simulink model "p3"  (R2020b)
settings: Solver=VariableStepAuto  StartTime=0.0  StopTime=5  RelTol=1e-3
undefined symbols (not defined in the file): A, A1, B, B1, C, C1, K, K1, KDelay
libraries: simulink x2
settings Model: Creator=Julian  LastModifiedBy=Julian

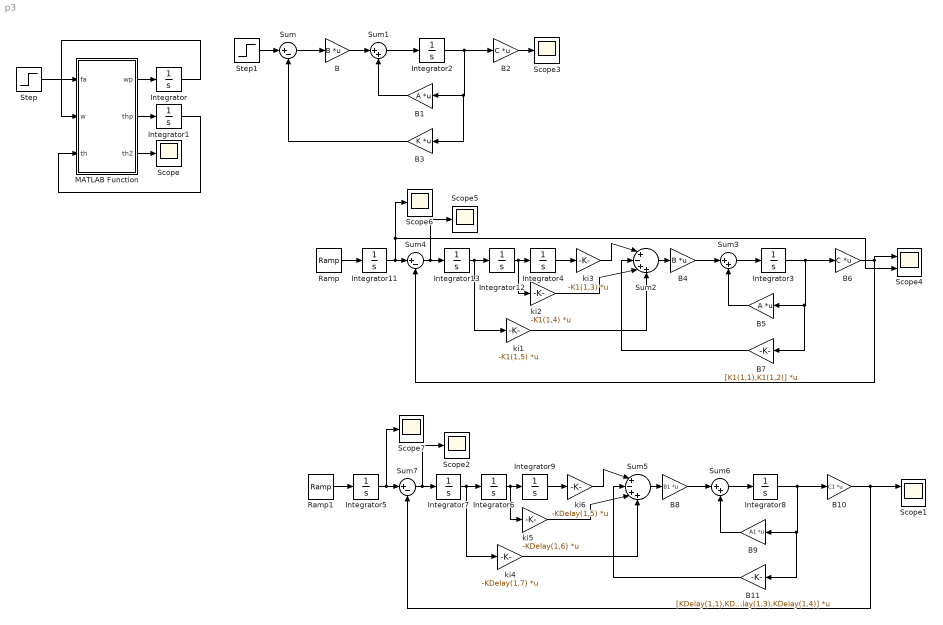
== system p3 ==
  B : Gain  Gain=B  Multiplication=Matrix(K*u)
  B1 : Gain  Gain=A  Multiplication=Matrix(K*u)
  B10 : Gain  Gain=C1  Multiplication=Matrix(K*u)
  B11 : Gain  Gain=[KDelay(1,1),KDelay(1,2),KDelay(1,3),KDelay(1,4)]  Multiplication=Matrix(K*u)
  B2 : Gain  Gain=C  Multiplication=Matrix(K*u)
  B3 : Gain  Gain=K  Multiplication=Matrix(K*u)
  B4 : Gain  Gain=B  Multiplication=Matrix(K*u)
  B5 : Gain  Gain=A  Multiplication=Matrix(K*u)
  B6 : Gain  Gain=C  Multiplication=Matrix(K*u)
  B7 : Gain  Gain=[K1(1,1),K1(1,2)]  Multiplication=Matrix(K*u)
  B8 : Gain  Gain=B1  Multiplication=Matrix(K*u)
  B9 : Gain  Gain=A1  Multiplication=Matrix(K*u)
  Integrator{,1..9,11..13} (13 alike) : Integrator
  MATLAB Function : MATLAB Function  TreatAsAtomicUnit=on
  Ramp : simulink/Sources/Ramp  slope=0.5  start=0  InitialOutput=0
  Ramp1 : simulink/Sources/Ramp  slope=0.5  start=0.5  InitialOutput=0
  Scope{,2..3,5..7} (6 alike) : Scope
  Scope1 : Scope  NumInputPorts=2
  Scope4 : Scope  NumInputPorts=2
  Step : Step  Time=0  SampleTime=0
  Step1 : Step  Time=0  SampleTime=0
  Sum : Sum  Inputs=|+-
  Sum1 : Sum  Inputs=|++
  Sum2 : Sum  Inputs=|+-++
  Sum3 : Sum  Inputs=|++
  Sum4 : Sum  Inputs=|+-
  Sum5 : Sum  Inputs=|+-++
  Sum6 : Sum  Inputs=|++
  Sum7 : Sum  Inputs=|+-
  ki1 : Gain  Gain=-K1(1,5)  Multiplication=Matrix(K*u)
  ki2 : Gain  Gain=-K1(1,4)  Multiplication=Matrix(K*u)
  ki3 : Gain  Gain=-K1(1,3)  Multiplication=Matrix(K*u)
  ki4 : Gain  Gain=-KDelay(1,7)  Multiplication=Matrix(K*u)
  ki5 : Gain  Gain=-KDelay(1,6)  Multiplication=Matrix(K*u)
  ki6 : Gain  Gain=-KDelay(1,5)  Multiplication=Matrix(K*u)
  wires:
  MATLAB Function/1(wp) -> Integrator/1
  MATLAB Function/2(thp) -> Integrator1/1
  Integrator/1 -> MATLAB Function/2(w)
  Integrator1/1 -> MATLAB Function/3(th)
  Step/1 -> MATLAB Function/1(fa)
  MATLAB Function/3(th2) -> Scope/1
  Integrator2/1 -> B2/1, B3/1, B1/1
  B2/1 -> Scope3/1
  Step1/1 -> Sum/1
  B/1 -> Sum1/1
  Sum/1 -> B/1
  B1/1 -> Sum1/2
  B3/1 -> Sum/2
  Sum1/1 -> Integrator2/1
  B4/1 -> Sum3/1
  Integrator4/1 -> ki3/1
  B5/1 -> Sum3/2
  B6/1 -> Sum4/2, Scope4/1
  ki3/1 -> Sum2/1
  Sum2/1 -> B4/1
  Integrator3/1 -> B6/1, B7/1, B5/1
  B7/1 -> Sum2/2
  Sum3/1 -> Integrator3/1
  Integrator11/1 -> Scope4/2, Scope6/1, Sum4/1
  Sum4/1 -> Scope5/1, Integrator13/1
  Integrator13/1 -> ki1/1, Integrator12/1
  Integrator12/1 -> ki2/1, Integrator4/1
  ki2/1 -> Sum2/3
  ki1/1 -> Sum2/4
  Ramp/1 -> Integrator11/1
  Ramp1/1 -> Integrator5/1
  ki4/1 -> Sum5/4
  B9/1 -> Sum6/2
  Integrator5/1 -> Scope7/1, Sum7/1
  Sum6/1 -> Integrator8/1
  ki5/1 -> Sum5/3
  B8/1 -> Sum6/1
  Integrator7/1 -> ki4/1, Integrator6/1
  Integrator8/1 -> B10/1, B11/1, B9/1
  B11/1 -> Sum5/2
  ki6/1 -> Sum5/1
  Sum7/1 -> Scope2/1, Integrator7/1
  Integrator6/1 -> ki5/1, Integrator9/1
  Sum5/1 -> B8/1
  Integrator9/1 -> ki6/1
  B10/1 -> Scope1/1, Sum7/2

== matlab function p3/MATLAB Function ==
  data: fa input; wp output; w input; th input; thp output; th2 output
function [wp,thp,th2] = fcn(fa,w,th)
J=0.01;
r=0.1;
r2=r/2;
k=1;
k2=0.5;
b=0.1;
g=9.81;
m=1;

thp=w;
wp=(1/(J+m*r*r))*(r*(fa+m*g)-b*w-k*r*r*th-((r*r)/(r2*r2))*k2*th);
th2=(r/r2)*th;
